simulink model "smc_diff_update"  (R2024b)
settings: Solver=ode1  StartTime=0.0  StopTime=15  FixedStep=1e-5  RelTol=1e-3
libraries: simulink x1
settings Model: Creator=user  LastModifiedBy=user

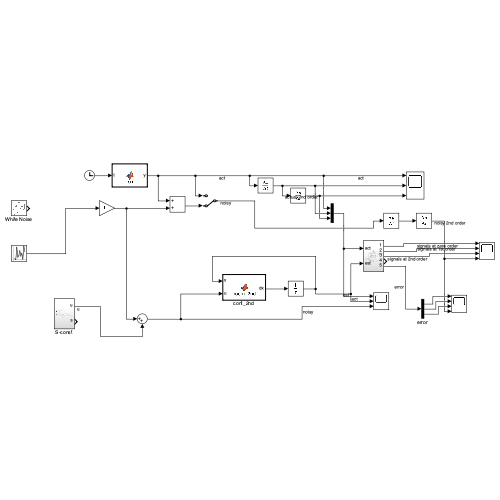
[thumbnail: Simulink's stored preview of the top-level diagram]
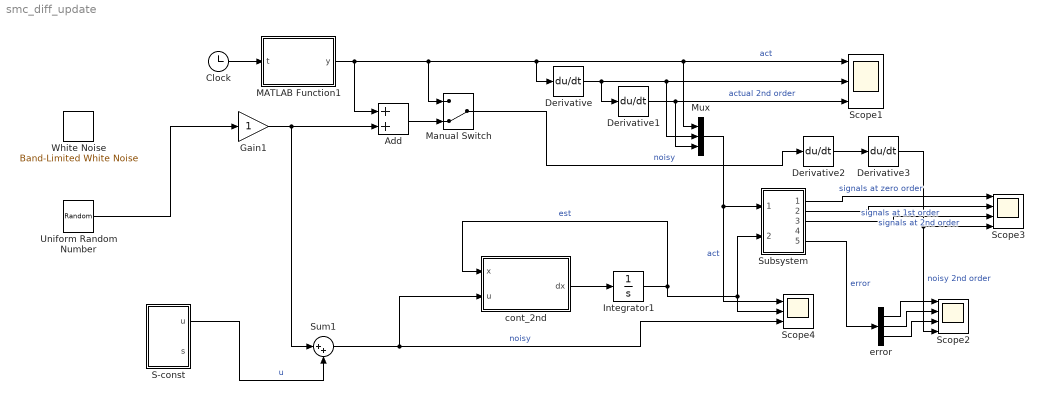
== system smc_diff_update ==
  Add : Sum
  Clock : Clock
  Derivative{,1..3} (4 alike) : Derivative
  Gain1 : Gain
  Integrator1 : Integrator
  MATLAB Function1 : MATLAB Function  TreatAsAtomicUnit=on
  Manual Switch : ManualSwitch  CurrentSetting=0
  Mux : Mux  Inputs=3
  S-const : Subsystem
  Scope1 : Scope  NumInputPorts=3
  Scope2 : Scope  NumInputPorts=4
  Scope3 : Scope  NumInputPorts=4
  Scope4 : Scope  NumInputPorts=3
  Subsystem : Subsystem
  Sum1 : Sum  Inputs=|++
  Uniform Random Number : UniformRandomNumber  Minimum=-1e-3  Maximum=1e-3  SampleTime=0.001
  White Noise : simulink/Sources/Band-Limited White Noise  Cov=1e-8*0  Ts=0.001  seed=[23341]
  cont_2nd : MATLAB Function  TreatAsAtomicUnit=on
  error : Demux  Outputs=3
  wires:
  Clock/1 -> MATLAB Function1/1(t)
  Derivative/1 -> Scope1/2, Mux/2, Derivative1/1
  Derivative1/1 -> Scope1/3, Mux/3  "actual 2nd order"
  Mux/1 -> Scope4/1, Subsystem/1(act)  "act"
  cont_2nd/1(dx) -> Integrator1/1
  Integrator1/1 -> cont_2nd/1(x), Scope4/2, Subsystem/2(est)  "est"
  Sum1/1 -> Scope4/3, cont_2nd/2(u)  "noisy"
  Add/1 -> Manual Switch/2
  MATLAB Function1/1(y) -> Derivative/1, Mux/1, Scope1/1, Manual Switch/1, Add/1  "act"
  Manual Switch/1 -> Derivative2/1  "noisy"
  S-const/1(u) -> Sum1/2  "u"
  Subsystem/1(Out1) -> Scope3/1  "signals at zero order"
  Subsystem/2(Out2) -> Scope3/2  "signals at 1st order"
  Subsystem/3(Out3) -> Scope3/3  "signals at 2nd order"
  Derivative2/1 -> Derivative3/1
  Gain1/1 -> Sum1/1, Add/2
  Subsystem/5(Out5) -> error/1  "error"
  error/1 -> Scope2/1
  error/2 -> Scope2/2
  error/3 -> Scope2/3
  Derivative3/1 -> Scope3/4, Scope2/4  "noisy 2nd order"
  Uniform Random Number/1 -> Gain1/1

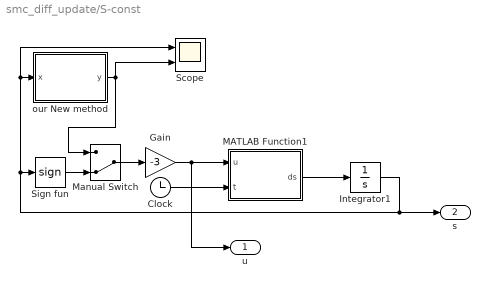
== system smc_diff_update/S-const ==
  Clock : Clock
  Gain : Gain  Gain=-3
  Integrator1 : Integrator  InitialCondition=5
  MATLAB Function1 : MATLAB Function  TreatAsAtomicUnit=on
  Manual Switch : ManualSwitch  CurrentSetting=0
  Scope : Scope  NumInputPorts=2
  Sign fun : Signum
  "our New method " : MATLAB Function  TreatAsAtomicUnit=on
  u : Outport
  s : Outport  Port=2
  wires:
  MATLAB Function1/1(ds) -> Integrator1/1
  Integrator1/1 -> Sign fun/1, Scope/1, "our New method "/1(x), s/1
  Clock/1 -> MATLAB Function1/2(t)
  Gain/1 -> MATLAB Function1/1(u), u/1
  "our New method "/1(y) -> Manual Switch/1, Scope/2
  Sign fun/1 -> Manual Switch/2
  Manual Switch/1 -> Gain/1

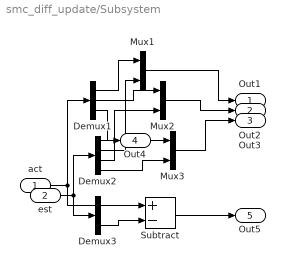
== system smc_diff_update/Subsystem ==
  act : Inport
  est : Inport  Port=2
  Demux1 : Demux  Outputs=3
  Demux2 : Demux  Outputs=[2 1 1 1]
  Demux3 : Demux  Outputs=[2, 3]
  Mux1 : Mux  Inputs=2
  Mux2 : Mux  Inputs=2
  Mux3 : Mux  Inputs=2
  Subtract : Sum  Inputs=+-
  Out1 : Outport
  Out2 : Outport  Port=2
  Out3 : Outport  Port=3
  Out4 : Outport  Port=4
  Out5 : Outport  Port=5
  wires:
  act/1 -> Subtract/1, Demux1/1
  Demux1/2 -> Mux2/1
  Mux3/1 -> Out3/1
  Demux2/1 -> Out4/1
  Demux1/1 -> Mux1/1
  Demux2/4 -> Mux3/2
  Mux1/1 -> Out1/1
  Demux2/2 -> Mux1/2
  est/1 -> Demux3/1, Demux2/1
  Mux2/1 -> Out2/1
  Demux1/3 -> Mux3/1
  Demux2/3 -> Mux2/2
  Subtract/1 -> Out5/1
  Demux3/2 -> Subtract/2

== matlab function smc_diff_update/S-const/MATLAB Function1 ==
  data: u input; ds output; t input
function ds = fcn(u, t)
    ds = cos(t) + (2 + sin(3*t))*u;
    %ds = (1+exp(-2*t))*sin(2*t) + (5 + cos(t))*u;
end

== matlab function smc_diff_update/MATLAB Function1 ==
  data: t input; y output
function y = fcn(t)

y = -cos(t)/(2+sin(3*t));
%y = -(1+exp(-2*t))*sin(2*t)/(5+cos(t));

== matlab function smc_diff_update/S-const/our New method  ==
  data: x input; y output
% function y = bisigmoid(x)
%     k = 1e4; c = 1;
%     y = tanh(k * x);
% end

function y = alevantbook(x)

  y = x/(abs(x)+1e-8);

end

== matlab function smc_diff_update/cont_2nd ==
  data: x input; u input; dx output
function dx = hosm_2nd(x, u)

dx = zeros(5, 1);
% OUTPUT:
%   dx     - derivative of state vector (5x1)
L = 35;
gamma = 1;
lambda = [1.1 3.06, 4.16 3];
k = length(lambda) - 1;  
% Extract states for clarity:
z_m2 = x(1);   % z_{-2}
z_m1 = x(2);   % z_{-1}
z0   = x(3);   % z_0, estimate of u_eq
z1   = x(4);   % z_1, estimate of u_eq derivative
z2   = x(5);   % z_2, estimate of u_eq second derivative

% Extract lambda parameters:
lambda0 = lambda(1);
lambda1 = lambda(2);
lambda2 = lambda(3);
lambda3 = lambda(4);

% Compute the error term for the differentiator.
% Here the error is defined as e = z_m1 - z_m2.
e = z_m1 - z_m2;

% Define the fractional power function:
% fpower(w, alpha) = |w|^alpha * sign(w)
fpower = @(w, alpha) (abs(w)^alpha) * sign(w);

dz_m2 = u - gamma * z_m2;
dz_m1 = -lambda3 * L^(1/4) * fpower(e, 3/4) + z0 - gamma * z_m2;
dz0   = -lambda2 * L^(2/4) * fpower(e, 2/4) + z1;
dz1   = -lambda1 * L^(3/4) * fpower(e, 1/4) + z2;
dz2   = -lambda0 * L * sign(e);

%-----------------------------------------------------------------------
% Assemble the state derivative vector:
dx = [dz_m2; dz_m1; dz0; dz1; dz2];

end
